simulink model "gm_parallel_8_prediction"  (R2022a)
settings: Solver=FixedStepDiscrete  StartTime=0.0  StopTime=10.0  RelTol=1e-3
undefined symbols (not defined in the file or in its folder): f_c, L_d, L_q, L_x, L_y, p, psi_pm, R_ph
libraries: hdlmdlgenlib x2
(part 1 of 4)
settings Model: Creator=Andre Merx  LastModifiedBy=Andre Merx
settings SolverCC: AlgebraicLoopSolver=TrustRegion
settings DataIOCC: LimitDataPoints=on  SaveOutput=off  SaveTime=off
settings OptimizationCC: BlockReduction=off  ConditionallyExecuteInputs=off  DefaultParameterBehavior=Inlined  LifeSpan=inf
settings DebuggingCC: AlgebraicLoopMsg=error  InheritedTsInSrcMsg=none  SingleTaskRateTransMsg=error  UnconnectedInputMsg=warning  UnconnectedOutputMsg=warning  UnconnectedLineMsg=warning  AllowSymbolicDim=off  StrictBusMsg=ErrorOnBusTreatedAsVector  SFUnexpectedBacktrackingDiag=warning  SFNoUnconditionalDefaultTransitionDiag=warning  SFExecutionAtInitializationDiag=none  SFMachineParentedDataDiag=warning  ArithmeticOperatorsInVariantConditions=warning
settings HardwareCC: ProdBitPerPointer=32  ProdBitPerSizeT=32  ProdBitPerPtrDiffT=32  ProdLargestAtomicFloat=None  ProdIntDivRoundTo=Undefined  ProdEndianess=Unspecified  ProdWordSize=32  ProdHWDeviceType=ASIC/FPGA->ASIC/FPGA  ProdEqTarget=off
settings SFSimCC: SimUseLocalCustomCode=off  CustomCodeUndefinedFunction=UseInterfaceOnly
settings RTWCC: RTWUseLocalCustomCode=off
settings CodeAppCC: StateflowObjectComments=on
settings GRTTargetCC: TargetLangStandard=C89/C90 (ANSI)
settings ConfigComp: CovScope=ReferencedModels  CovMetricSettings=dw  CovSaveCumulativeToWorkspaceVar=on  CovSaveSingleToWorkspaceVar=on  CovExternalEMLEnable=off  CovSFcnEnable=off

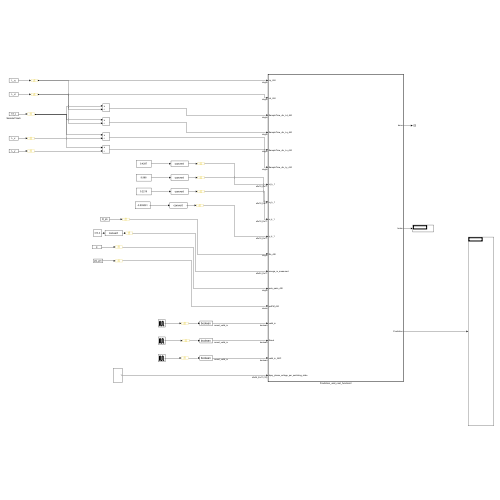
[thumbnail: Simulink's stored preview of the top-level diagram]
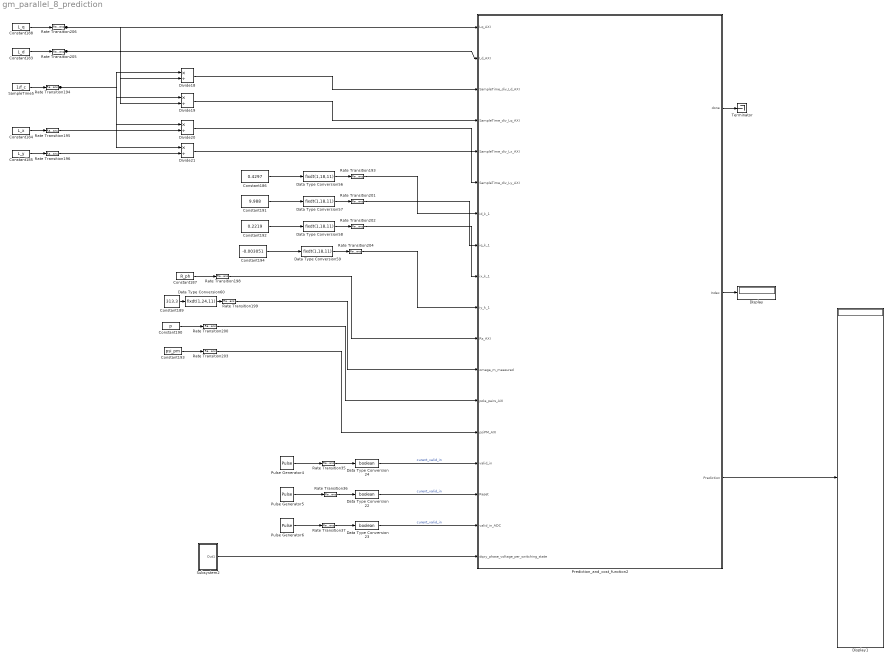
== system gm_parallel_8_prediction ==
  Constant183 : Constant  Value=L_d  OutDataTypeStr=single  SampleTime=-1
  Constant184 : Constant  Value=L_x  OutDataTypeStr=single  SampleTime=-1
  Constant185 : Constant  Value=L_y  OutDataTypeStr=single  SampleTime=-1
  Constant186 : Constant  Value=0.4297
  Constant187 : Constant  Value=R_ph  OutDataTypeStr=single  SampleTime=-1
  Constant188 : Constant  Value=L_q  OutDataTypeStr=single  SampleTime=-1
  Constant189 : Constant  Value=313.3
  Constant190 : Constant  Value=p  OutDataTypeStr=single  SampleTime=-1
  Constant191 : Constant  Value=9.988
  Constant192 : Constant  Value=0.2219
  Constant193 : Constant  Value=psi_pm  OutDataTypeStr=single  SampleTime=-1
  Constant194 : Constant  Value=-0.003051
  Data Type Conversion22 : DataTypeConversion  OutDataTypeStr=boolean  SaturateOnIntegerOverflow=off  RndMeth=Floor
  Data Type Conversion23 : DataTypeConversion  OutDataTypeStr=boolean  SaturateOnIntegerOverflow=off  RndMeth=Floor
  Data Type Conversion24 : DataTypeConversion  OutDataTypeStr=boolean  SaturateOnIntegerOverflow=off  RndMeth=Floor
  Data Type Conversion{56..59} (4 alike) : DataTypeConversion  OutDataTypeStr=fixdt(1,18,11)  SaturateOnIntegerOverflow=off  RndMeth=Floor
  Data Type Conversion60 : DataTypeConversion  OutDataTypeStr=fixdt(1,24,11)  SaturateOnIntegerOverflow=off  RndMeth=Floor
  Display : Display
  Display1 : Display
  Divide{18..21} (4 alike) : Product  Inputs=*/  RndMeth=Zero  SaturateOnIntegerOverflow=on
  Prediction_and_cost_function2 : Subsystem  TreatAsAtomicUnit=on
  Pulse Generator4 : DiscretePulseGenerator  PulseType=Time based  Period=1/f_c
  Pulse Generator5 : DiscretePulseGenerator  PulseType=Time based  Period=1/f_c
  Pulse Generator6 : DiscretePulseGenerator  PulseType=Time based  Period=1/f_c
  Rate Transition{35..37,193..196,198..206} (16 alike) : RateTransition  OutPortSampleTime=Rt
  SampleTime5 : Constant  Value=1/f_c  OutDataTypeStr=single  SampleTime=-1
  Subsystem2 : Subsystem
  Terminator : Terminator
  wires:
  Prediction_and_cost_function2/3(Prediction) -> Display1/1
  Prediction_and_cost_function2/2(Index) -> Display/1
  Prediction_and_cost_function2/1(done) -> Terminator/1
  Pulse Generator5/1 -> Rate Transition36/1
  Pulse Generator6/1 -> Rate Transition37/1
  Data Type Conversion22/1 -> Prediction_and_cost_function2/16(Reset)  "curent_valid_in"
  Data Type Conversion24/1 -> Prediction_and_cost_function2/15(valid_in)  "curent_valid_in"
  Rate Transition37/1 -> Data Type Conversion23/1
  Rate Transition35/1 -> Data Type Conversion24/1
  Data Type Conversion23/1 -> Prediction_and_cost_function2/17(valid_in_ADC)  "curent_valid_in"
  Rate Transition36/1 -> Data Type Conversion22/1
  Pulse Generator4/1 -> Rate Transition35/1
  Rate Transition204/1 -> Prediction_and_cost_function2/10(iy_k_1)
  Rate Transition193/1 -> Prediction_and_cost_function2/7(id_k_1)
  Rate Transition194/1 -> Divide18/1, Divide20/1, Divide21/1, Divide19/1
  Rate Transition198/1 -> Prediction_and_cost_function2/11(Rs_AXI)
  Divide18/1 -> Prediction_and_cost_function2/3(SampleTime_div_Ld_AXI)
  Constant191/1 -> Data Type Conversion57/1
  Constant185/1 -> Rate Transition196/1
  Rate Transition202/1 -> Prediction_and_cost_function2/9(ix_k_1)
  Divide21/1 -> Prediction_and_cost_function2/6(SampleTime_div_Ly_AXI)
  Constant189/1 -> Data Type Conversion60/1
  Constant183/1 -> Rate Transition205/1
  Constant184/1 -> Rate Transition195/1
  Constant193/1 -> Rate Transition203/1
  Rate Transition200/1 -> Prediction_and_cost_function2/13(pole_pairs_AXI)
  Rate Transition206/1 -> Prediction_and_cost_function2/1(Lq_AXI), Divide19/2
  Divide19/1 -> Prediction_and_cost_function2/4(SampleTime_div_Lq_AXI)
  Rate Transition196/1 -> Divide21/2
  Constant192/1 -> Data Type Conversion58/1
  Data Type Conversion56/1 -> Rate Transition193/1
  Rate Transition203/1 -> Prediction_and_cost_function2/14(psiPM_AXI)
  Constant187/1 -> Rate Transition198/1
  Divide20/1 -> Prediction_and_cost_function2/5(SampleTime_div_Lx_AXI)
  Data Type Conversion57/1 -> Rate Transition201/1
  Constant186/1 -> Data Type Conversion56/1
  SampleTime5/1 -> Rate Transition194/1
  Rate Transition195/1 -> Divide20/2
  Data Type Conversion58/1 -> Rate Transition202/1
  Rate Transition205/1 -> Prediction_and_cost_function2/2(Ld_AXI), Divide18/2
  Subsystem2/1(Out1) -> Prediction_and_cost_function2/18(dqxy_phase_voltage_per_switching_state)
  Constant190/1 -> Rate Transition200/1
  Data Type Conversion59/1 -> Rate Transition204/1
  Rate Transition201/1 -> Prediction_and_cost_function2/8(iq_k_1)
  Constant188/1 -> Rate Transition206/1
  Constant194/1 -> Data Type Conversion59/1
  Rate Transition199/1 -> Prediction_and_cost_function2/12(omega_m_measured)
  Data Type Conversion60/1 -> Rate Transition199/1

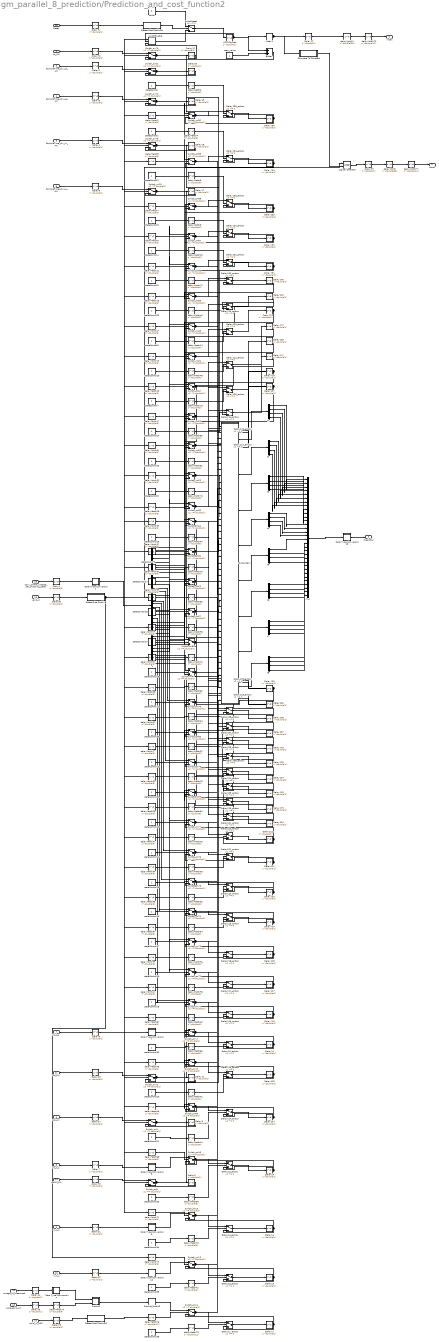
== system gm_parallel_8_prediction/Prediction_and_cost_function2 ==
  Lq_AXI : Inport  OutDataTypeStr=single  PortDimensions=1  SampleTime=1e-08
  Ld_AXI : Inport  Port=2  OutDataTypeStr=single  PortDimensions=1  SampleTime=1e-08
  SampleTime_div_Ld_AXI : Inport  Port=3  OutDataTypeStr=single  PortDimensions=1  SampleTime=1e-08
  SampleTime_div_Lq_AXI : Inport  Port=4  OutDataTypeStr=single  PortDimensions=1  SampleTime=1e-08
  SampleTime_div_Lx_AXI : Inport  Port=5  OutDataTypeStr=single  PortDimensions=1  SampleTime=1e-08
  SampleTime_div_Ly_AXI : Inport  Port=6  OutDataTypeStr=single  PortDimensions=1  SampleTime=1e-08
  id_k_1 : Inport  Port=7  OutDataTypeStr=fixdt(1, 18, 11)  PortDimensions=1  SampleTime=1e-08
  iq_k_1 : Inport  Port=8  OutDataTypeStr=fixdt(1, 18, 11)  PortDimensions=1  SampleTime=1e-08
  ix_k_1 : Inport  Port=9  OutDataTypeStr=fixdt(1, 18, 11)  PortDimensions=1  SampleTime=1e-08
  iy_k_1 : Inport  Port=10  OutDataTypeStr=fixdt(1, 18, 11)  PortDimensions=1  SampleTime=1e-08
  Rs_AXI : Inport  Port=11  OutDataTypeStr=single  PortDimensions=1  SampleTime=1e-08
  omega_m_measured : Inport  Port=12  OutDataTypeStr=fixdt(1, 24, 11)  PortDimensions=1  SampleTime=1e-08
  pole_pairs_AXI : Inport  Port=13  OutDataTypeStr=single  PortDimensions=1  SampleTime=1e-08
  psiPM_AXI : Inport  Port=14  OutDataTypeStr=single  PortDimensions=1  SampleTime=1e-08
  valid_in : Inport  Port=15  OutDataTypeStr=boolean  PortDimensions=1  SampleTime=1e-08
  Reset : Inport  Port=16  OutDataTypeStr=boolean  PortDimensions=1  SampleTime=1e-08
  valid_in_ADC : Inport  Port=17  OutDataTypeStr=boolean  PortDimensions=1  SampleTime=1e-08
  dqxy_phase_voltage_per_switching_state : Inport  Port=18  OutDataTypeStr=fixdt(1, 24, 11)  PortDimensions=[32]  SampleTime=1e-08
  Compare To Constant : Subsystem  mask(Compare To Constant){relop=<=, const=double(8), OutDataTypeStr=boolean, ZeroCross=on}
      mask prompts: relop "Simulink:masks:Operator_MP"; const "Simulink:masks:ConstantValue_MP"; OutDataTypeStr "Simulink:masks:OutputDataType_MP"; ZeroCross "Simulink:masks:EnableZerocrossingDetection_MP"
      mask help: Simulink:masks:CompareToConstant_MD
      mask init:
      | OutDataTypeStr = 'boolean';
      | ZeroCross = 'on';
      | blkName = 'parallel_8_prediction/Prediction_and_cost_function2/Compare\nTo Constant';
      | const = double(8);
      | const_str = '8';
      | const_val = double(8);
      | relop = '<=';
      | setValue = 'boolean';
      | str = '<= 8';
      mask TypeOptions relop: == | ~= | < | <= | >= | >
      mask TypeOptions OutDataTypeStr: Simulink:masks:uint8 | Simulink:masks:boolean
      mask Callback ZeroCross: sl('zeroCrossEnable', gcbh);
      mask Display: disp(str)
  Data Type Conversion1 : Subsystem
      mask Display: disp('NFP\nconv');
  Data Type Conversion10 : Subsystem
      mask Display: disp('NFP\nconv');
  Data Type Conversion18 : Subsystem
      mask Display: disp('NFP\nconv');
  Data Type Conversion4 : Subsystem
      mask Display: disp('NFP\nconv');
  Data Type Conversion7 : Subsystem
      mask Display: disp('NFP\nconv');
  Data Type Conversion8 : Subsystem
      mask Display: disp('NFP\nconv');
  Data Type Conversion9 : Subsystem
      mask Display: disp('NFP\nconv');
  Delay{1..33,104..135} (65 alike) : Delay  DelayLength=double(1)  InitialCondition=0  SampleTime=1e-08
  Delay104_enbsw : Switch  Criteria=u2 ~= 0  Threshold=double(0)  OutDataTypeStr=single  SampleTime=1e-08  SaturateOnIntegerOverflow=off  InputSameDT=off
  Delay105_enbsw : Switch  Criteria=u2 ~= 0  Threshold=double(0)  OutDataTypeStr=single  SampleTime=1e-08  SaturateOnIntegerOverflow=off  InputSameDT=off
  Delay106_enbsw : Switch  Criteria=u2 ~= 0  Threshold=double(0)  OutDataTypeStr=single  SampleTime=1e-08  SaturateOnIntegerOverflow=off  InputSameDT=off
  Delay107_enbsw : Switch  Criteria=u2 ~= 0  Threshold=double(0)  OutDataTypeStr=single  SampleTime=1e-08  SaturateOnIntegerOverflow=off  InputSameDT=off
  Delay108_enbsw : Switch  Criteria=u2 ~= 0  Threshold=double(0)  OutDataTypeStr=single  SampleTime=1e-08  SaturateOnIntegerOverflow=off  InputSameDT=off
  Delay109_enbsw : Switch  Criteria=u2 ~= 0  Threshold=double(0)  OutDataTypeStr=single  SampleTime=1e-08  SaturateOnIntegerOverflow=off  InputSameDT=off
  Delay110_enbsw : Switch  Criteria=u2 ~= 0  Threshold=double(0)  OutDataTypeStr=single  SampleTime=1e-08  SaturateOnIntegerOverflow=off  InputSameDT=off
  Delay111_enbsw : Switch  Criteria=u2 ~= 0  Threshold=double(0)  OutDataTypeStr=single  SampleTime=1e-08  SaturateOnIntegerOverflow=off  InputSameDT=off
  Delay112_enbsw : Switch  Criteria=u2 ~= 0  Threshold=double(0)  OutDataTypeStr=single  SampleTime=1e-08  SaturateOnIntegerOverflow=off  InputSameDT=off
  Delay113_enbsw : Switch  Criteria=u2 ~= 0  Threshold=double(0)  OutDataTypeStr=single  SampleTime=1e-08  SaturateOnIntegerOverflow=off  InputSameDT=off
  Delay114_enbsw : Switch  Criteria=u2 ~= 0  Threshold=double(0)  OutDataTypeStr=single  SampleTime=1e-08  SaturateOnIntegerOverflow=off  InputSameDT=off
  Delay115_enbsw : Switch  Criteria=u2 ~= 0  Threshold=double(0)  OutDataTypeStr=single  SampleTime=1e-08  SaturateOnIntegerOverflow=off  InputSameDT=off
  Delay116_enbsw : Switch  Criteria=u2 ~= 0  Threshold=double(0)  OutDataTypeStr=single  SampleTime=1e-08  SaturateOnIntegerOverflow=off  InputSameDT=off
  Delay117_enbsw : Switch  Criteria=u2 ~= 0  Threshold=double(0)  OutDataTypeStr=single  SampleTime=1e-08  SaturateOnIntegerOverflow=off  InputSameDT=off
  Delay118_enbsw : Switch  Criteria=u2 ~= 0  Threshold=double(0)  OutDataTypeStr=single  SampleTime=1e-08  SaturateOnIntegerOverflow=off  InputSameDT=off
  Delay119_enbsw : Switch  Criteria=u2 ~= 0  Threshold=double(0)  OutDataTypeStr=single  SampleTime=1e-08  SaturateOnIntegerOverflow=off  InputSameDT=off
  Delay11_enbsw : Switch  Criteria=u2 ~= 0  Threshold=double(0)  OutDataTypeStr=single  SampleTime=1e-08  SaturateOnIntegerOverflow=off  InputSameDT=off
  Delay120_enbsw : Switch  Criteria=u2 ~= 0  Threshold=double(0)  OutDataTypeStr=single  SampleTime=1e-08  SaturateOnIntegerOverflow=off  InputSameDT=off
  Delay121_enbsw : Switch  Criteria=u2 ~= 0  Threshold=double(0)  OutDataTypeStr=single  SampleTime=1e-08  SaturateOnIntegerOverflow=off  InputSameDT=off
  Delay122_enbsw : Switch  Criteria=u2 ~= 0  Threshold=double(0)  OutDataTypeStr=single  SampleTime=1e-08  SaturateOnIntegerOverflow=off  InputSameDT=off
  Delay123_enbsw : Switch  Criteria=u2 ~= 0  Threshold=double(0)  OutDataTypeStr=single  SampleTime=1e-08  SaturateOnIntegerOverflow=off  InputSameDT=off
  Delay124_enbsw : Switch  Criteria=u2 ~= 0  Threshold=double(0)  OutDataTypeStr=single  SampleTime=1e-08  SaturateOnIntegerOverflow=off  InputSameDT=off
  Delay125_enbsw : Switch  Criteria=u2 ~= 0  Threshold=double(0)  OutDataTypeStr=single  SampleTime=1e-08  SaturateOnIntegerOverflow=off  InputSameDT=off
  Delay126_enbsw : Switch  Criteria=u2 ~= 0  Threshold=double(0)  OutDataTypeStr=single  SampleTime=1e-08  SaturateOnIntegerOverflow=off  InputSameDT=off
  Delay127_enbsw : Switch  Criteria=u2 ~= 0  Threshold=double(0)  OutDataTypeStr=single  SampleTime=1e-08  SaturateOnIntegerOverflow=off  InputSameDT=off
  Delay128_enbsw : Switch  Criteria=u2 ~= 0  Threshold=double(0)  OutDataTypeStr=single  SampleTime=1e-08  SaturateOnIntegerOverflow=off  InputSameDT=off
  Delay129_enbsw : Switch  Criteria=u2 ~= 0  Threshold=double(0)  OutDataTypeStr=single  SampleTime=1e-08  SaturateOnIntegerOverflow=off  InputSameDT=off
  Delay130_enbsw : Switch  Criteria=u2 ~= 0  Threshold=double(0)  OutDataTypeStr=single  SampleTime=1e-08  SaturateOnIntegerOverflow=off  InputSameDT=off
  Delay131_enbsw : Switch  Criteria=u2 ~= 0  Threshold=double(0)  OutDataTypeStr=single  SampleTime=1e-08  SaturateOnIntegerOverflow=off  InputSameDT=off
  Delay132_enbsw : Switch  Criteria=u2 ~= 0  Threshold=double(0)  OutDataTypeStr=single  SampleTime=1e-08  SaturateOnIntegerOverflow=off  InputSameDT=off
  Delay133_enbsw : Switch  Criteria=u2 ~= 0  Threshold=double(0)  OutDataTypeStr=single  SampleTime=1e-08  SaturateOnIntegerOverflow=off  InputSameDT=off
  Delay134_enbsw : Switch  Criteria=u2 ~= 0  Threshold=double(0)  OutDataTypeStr=single  SampleTime=1e-08  SaturateOnIntegerOverflow=off  InputSameDT=off
  Delay135_enbsw : Switch  Criteria=u2 ~= 0  Threshold=double(0)  OutDataTypeStr=single  SampleTime=1e-08  SaturateOnIntegerOverflow=off  InputSameDT=off
  Delay13_enbsw : Switch  Criteria=u2 ~= 0  Threshold=double(0)  OutDataTypeStr=single  SampleTime=1e-08  SaturateOnIntegerOverflow=off  InputSameDT=off
  Delay14_enbsw : Switch  Criteria=u2 ~= 0  Threshold=double(0)  OutDataTypeStr=single  SampleTime=1e-08  SaturateOnIntegerOverflow=off  InputSameDT=off
  Delay15_enbsw : Switch  Criteria=u2 ~= 0  Threshold=double(0)  OutDataTypeStr=single  SampleTime=1e-08  SaturateOnIntegerOverflow=off  InputSameDT=off
  Delay16_enbsw : Switch  Criteria=u2 ~= 0  Threshold=double(0)  OutDataTypeStr=single  SampleTime=1e-08  SaturateOnIntegerOverflow=off  InputSameDT=off
  Detect Rise Positive : Subsystem  mask(Detect Rise Positive){vinit=double(0), InputProcessing=Elements as channels (sample based), OutDataTypeStr=boolean}
      mask prompts: vinit "Simulink:masks:InitialCondition_MP"; InputProcessing "Simulink:masks:InputProcessing_MP"; OutDataTypeStr "Simulink:masks:OutputDataType_MP"
      mask help: Simulink:masks:DetectRisePositive_MD
      mask init:
      | InputProcessing = 'Elements as channels (sample based)';
      | OutDataTypeStr = 'boolean';
      | vinit = double(0);
      mask TypeOptions InputProcessing: Simulink:masks:ColumnsAsChannelsFrameBased | Simulink:masks:ElementsAsChannelsSampleBased
      mask TypeOptions OutDataTypeStr: Simulink:masks:uint8 | Simulink:masks:boolean
      mask Display: fprintf('U > 0\n&  NOT\nU/z > 0')
  Detect Rise Positive1 : Subsystem  mask(Detect Rise Positive){vinit=double(0), InputProcessing=Elements as channels (sample based), OutDataTypeStr=boolean}
      mask prompts: vinit "Simulink:masks:InitialCondition_MP"; InputProcessing "Simulink:masks:InputProcessing_MP"; OutDataTypeStr "Simulink:masks:OutputDataType_MP"
      mask help: Simulink:masks:DetectRisePositive_MD
      mask init:
      | InputProcessing = 'Elements as channels (sample based)';
      | OutDataTypeStr = 'boolean';
      | vinit = double(0);
      mask TypeOptions InputProcessing: Simulink:masks:ColumnsAsChannelsFrameBased | Simulink:masks:ElementsAsChannelsSampleBased
      mask TypeOptions OutDataTypeStr: Simulink:masks:uint8 | Simulink:masks:boolean
      mask Display: fprintf('U > 0\n&  NOT\nU/z > 0')
  Detect Rise Positive2 : Subsystem  mask(Detect Rise Positive){vinit=double(0), InputProcessing=Elements as channels (sample based), OutDataTypeStr=boolean}
      mask prompts: vinit "Simulink:masks:InitialCondition_MP"; InputProcessing "Simulink:masks:InputProcessing_MP"; OutDataTypeStr "Simulink:masks:OutputDataType_MP"
      mask help: Simulink:masks:DetectRisePositive_MD
      mask init:
      | InputProcessing = 'Elements as channels (sample based)';
      | OutDataTypeStr = 'boolean';
      | vinit = double(0);
      mask TypeOptions InputProcessing: Simulink:masks:ColumnsAsChannelsFrameBased | Simulink:masks:ElementsAsChannelsSampleBased
      mask TypeOptions OutDataTypeStr: Simulink:masks:uint8 | Simulink:masks:boolean
      mask Display: fprintf('U > 0\n&  NOT\nU/z > 0')
  HDL Counter : Delay  DelayLength=double(1)  InitialCondition=0  SampleTime=1e-08
  Index1 : hdlmdlgenlib/Buffer
      settings: SourceProductBaseCode=SL
  Logical Operator : Logic  AllPortsSameDT=off  OutDataTypeStr=boolean  SampleTime=1e-08
  Product : Subsystem
      mask Display: disp('NFP\nmul');
  Product_outbuff : hdlmdlgenlib/Buffer
      settings: SourceProductBaseCode=SL
  Subsystem : Subsystem
  Switch_on{8..13,15..21,59..90} (45 alike) : Switch  Threshold=double(1)  OutDataTypeStr=single  RndMeth=Simplest  SampleTime=1e-08  SaturateOnIntegerOverflow=off  InputSameDT=off
  adder : Sum  AccumDataTypeStr=int32  OutDataTypeStr=int32  SampleTime=1e-08
  const : Constant  Value=0  VectorParams1D=off  OutDataTypeStr=int32  SampleTime=1e-08
  delayMatch : Delay  DelayLength=double(36)  InitialCondition=0  SampleTime=1e-08
  delayMatch1 : Delay  DelayLength=double(36)  InitialCondition=0  SampleTime=1e-08
  delayMatch{2..74} (73 alike) : Delay  DelayLength=double(6)  InitialCondition=0  SampleTime=1e-08
  delayMatch75 : Delay  DelayLength=double(12)  InitialCondition=0  SampleTime=1e-08
  delayMatch76 : Delay  DelayLength=double(12)  InitialCondition=0  SampleTime=1e-08
  delayMatch77 : Delay  DelayLength=double(11)  InitialCondition=0  SampleTime=1e-08
  delayMatch78 : Delay  DelayLength=double(11)  InitialCondition=0  SampleTime=1e-08
  mux : Mux  Inputs=32
  stateControl{,1..36} (37 alike) : Constant  OutDataTypeStr=boolean  SampleTime=1e-08
  step_value : Constant  VectorParams1D=off  OutDataTypeStr=int32  SampleTime=1e-08
  switchEnable : MultiPortSwitch  DataPortOrder=Zero-based contiguous  Inputs=2  DiagnosticForDefault=None  zeroidx=on  OutDataTypeStr=int32  SampleTime=1e-08  SaturateOnIntegerOverflow=off  InputSameDT=off
  switchReset : Switch  Criteria=u2 ~= 0  Threshold=double(0)  OutDataTypeStr=int32  SampleTime=1e-08  SaturateOnIntegerOverflow=off  InputSameDT=off
  t : Demux  Outputs=32
  t{1..8} (8 alike) : Demux
  done : Outport  SampleTime=1e-08
  Index : Outport  Port=2  SampleTime=1e-08
  Prediction : Outport  Port=3  SampleTime=1e-08
  wires:
  Lq_AXI/1 -> Delay26/1
  Ld_AXI/1 -> Delay27/1
  SampleTime_div_Ld_AXI/1 -> Delay2/1
  SampleTime_div_Lq_AXI/1 -> Delay3/1
  SampleTime_div_Lx_AXI/1 -> Delay4/1
  SampleTime_div_Ly_AXI/1 -> Delay5/1
  id_k_1/1 -> Delay6/1
  iq_k_1/1 -> Delay7/1
  ix_k_1/1 -> Delay21/1
  iy_k_1/1 -> Delay22/1
  Rs_AXI/1 -> Delay23/1
  omega_m_measured/1 -> Delay24/1
  pole_pairs_AXI/1 -> Delay25/1
  psiPM_AXI/1 -> Delay28/1
  valid_in/1 -> Delay30/1
  Reset/1 -> Delay31/1
  valid_in_ADC/1 -> Delay29/1
  dqxy_phase_voltage_per_switching_state/1 -> Delay1/1
  Compare To Constant/1(y) -> Logical Operator/2
  Delay1/1 -> Data Type Conversion1/1(In1)
  Delay2/1 -> Switch_on21/1
  Delay21/1 -> Data Type Conversion9/1(In1)
  Delay22/1 -> Data Type Conversion10/1(In1)
  Delay23/1 -> Switch_on12/1
  Delay24/1 -> Data Type Conversion4/1(In1)
  delayMatch74/1 -> Product/2(In2)
  Delay26/1 -> Switch_on10/1
  Delay27/1 -> Switch_on9/1
  Delay28/1 -> Switch_on8/1
  Delay29/1 -> Detect Rise Positive2/1(U)
  Delay3/1 -> Switch_on20/1
  Delay30/1 -> Detect Rise Positive/1(U)
  Delay31/1 -> Detect Rise Positive1/1(U)
  delayMatch78/1 -> Index/1
  delayMatch77/1 -> done/1
  Delay4/1 -> Switch_on19/1
  Delay5/1 -> Switch_on18/1
  Delay6/1 -> Data Type Conversion7/1(In1)
  Delay7/1 -> Data Type Conversion8/1(In1)
  delayMatch3/1 -> Switch_on90/2
  Detect Rise Positive1/1(Y) -> switchReset/2
  delayMatch76/1 -> Switch_on11/2
  Index1/1 -> Delay32/1, Compare To Constant/1(u)
  Logical Operator/1 -> Delay33/1
  mux/1 -> Data Type Conversion18/1(In1)
  Product_outbuff/1 -> Switch_on11/1
  Subsystem/1(Prediction_1) -> t1/1
  Subsystem/2(Prediction_2) -> t2/1
  Subsystem/3(Prediction_3) -> t3/1
  Subsystem/4(Prediction_4) -> t4/1
  Subsystem/5(Prediction_5) -> t5/1
  Subsystem/6(Prediction_6) -> t6/1
  Subsystem/7(Prediction_7) -> t7/1
  Subsystem/8(Prediction_8) -> t8/1
  Switch_on10/1 -> Subsystem/43(Lq15), Delay10/1
  Switch_on12/1 -> Subsystem/41(Rs15), Delay12/1
  Switch_on18/1 -> Subsystem/36(SampleTime_div_Ly15), Delay17/1
  Switch_on19/1 -> Subsystem/35(SampleTime_div_Lx15), Delay18/1
  Switch_on20/1 -> Subsystem/34(SampleTime_div_Lq15), Delay19/1
  Switch_on21/1 -> Subsystem/33(SampleTime_div_Ld15), Delay20/1
  Switch_on8/1 -> Subsystem/45(psiPM15), Delay8/1
  Switch_on9/1 -> Subsystem/44(Ld15), Delay9/1
  HDL Counter/1 -> Index1/1, switchEnable/2, adder/1
  const/1 -> switchReset/1
  step_value/1 -> adder/2
  t/1 -> Switch_on90/1
  t/2 -> Switch_on89/1
  t/3 -> Switch_on88/1
  t/4 -> Switch_on87/1
  t/5 -> Switch_on86/1
  t/6 -> Switch_on85/1
  t/7 -> Switch_on84/1
  t/8 -> Switch_on83/1
  t/9 -> Switch_on82/1
  t/10 -> Switch_on81/1
  t/11 -> Switch_on80/1
  t/12 -> Switch_on79/1
  t/13 -> Switch_on78/1
  t/14 -> Switch_on77/1
  t/15 -> Switch_on76/1
  t/16 -> Switch_on75/1
  t/17 -> Switch_on74/1
  t/18 -> Switch_on73/1
  t/19 -> Switch_on72/1
  t/20 -> Switch_on71/1
  t/21 -> Switch_on70/1
  t/22 -> Switch_on69/1
  t/23 -> Switch_on68/1
  t/24 -> Switch_on67/1
  t/25 -> Switch_on66/1
  t/26 -> Switch_on65/1
  t/27 -> Switch_on64/1
  t/28 -> Switch_on63/1
  t/29 -> Switch_on62/1
  t/30 -> Switch_on61/1
  t/31 -> Switch_on60/1
  t/32 -> Switch_on59/1
  t1/1 -> mux/1
  t1/2 -> mux/2
  t1/3 -> mux/3
  t1/4 -> mux/4
  t2/1 -> mux/5
  t2/2 -> mux/6
  t2/3 -> mux/7
  t2/4 -> mux/8
  t3/1 -> mux/9
  t3/2 -> mux/10
  t3/3 -> mux/11
  t3/4 -> mux/12
  t4/1 -> mux/13
  t4/2 -> mux/14
  t4/3 -> mux/15
  t4/4 -> mux/16
  t5/1 -> mux/17
  t5/2 -> mux/18
  t5/3 -> mux/19
  t5/4 -> mux/20
  t6/1 -> mux/21
  t6/2 -> mux/22
  t6/3 -> mux/23
  t6/4 -> mux/24
  t7/1 -> mux/25
  t7/2 -> mux/26
  t7/3 -> mux/27
  t7/4 -> mux/28
  t8/1 -> mux/29
  t8/2 -> mux/30
  t8/3 -> mux/31
  t8/4 -> mux/32
  Delay33/1 -> delayMatch/1
  Delay32/1 -> delayMatch1/1
  Data Type Conversion1/1(Out1) -> t/1
  Data Type Conversion10/1(Out1) -> Switch_on13/1
  Data Type Conversion18/1(Out1) -> Prediction/1
  Data Type Conversion4/1(Out1) -> Product/1(In1)
  Data Type Conversion7/1(Out1) -> Switch_on17/1
  Data Type Conversion8/1(Out1) -> Switch_on16/1
  Data Type Conversion9/1(Out1) -> Switch_on15/1
  Product/1(Out1) -> Product_outbuff/1
  delayMatch2/1 -> Delay135_enbsw/2
  delayMatch4/1 -> Delay134_enbsw/2
  delayMatch6/1 -> Delay133_enbsw/2
  delayMatch8/1 -> Delay132_enbsw/2
  delayMatch10/1 -> Delay131_enbsw/2
  delayMatch12/1 -> Delay130_enbsw/2
  delayMatch14/1 -> Delay129_enbsw/2
  delayMatch16/1 -> Delay128_enbsw/2
  delayMatch18/1 -> Delay127_enbsw/2
  delayMatch20/1 -> Delay126_enbsw/2
  delayMatch22/1 -> Delay125_enbsw/2
  delayMatch24/1 -> Delay124_enbsw/2
  delayMatch26/1 -> Delay123_enbsw/2
  delayMatch28/1 -> Delay122_enbsw/2
  delayMatch30/1 -> Delay121_enbsw/2
  delayMatch32/1 -> Delay120_enbsw/2
  delayMatch34/1 -> Delay119_enbsw/2
  delayMatch36/1 -> Delay118_enbsw/2
  delayMatch38/1 -> Delay117_enbsw/2
  delayMatch40/1 -> Delay116_enbsw/2
  delayMatch42/1 -> Delay115_enbsw/2
  delayMatch44/1 -> Delay114_enbsw/2
  delayMatch46/1 -> Delay113_enbsw/2
  delayMatch48/1 -> Delay112_enbsw/2
  delayMatch50/1 -> Delay111_enbsw/2
  delayMatch52/1 -> Delay110_enbsw/2
  delayMatch54/1 -> Delay109_enbsw/2
  delayMatch56/1 -> Delay108_enbsw/2
  delayMatch58/1 -> Delay107_enbsw/2
  delayMatch60/1 -> Delay106_enbsw/2
  delayMatch62/1 -> Delay105_enbsw/2
  delayMatch64/1 -> Delay104_enbsw/2
  delayMatch66/1 -> Delay16_enbsw/2
  delayMatch68/1 -> Delay15_enbsw/2
  delayMatch70/1 -> Delay14_enbsw/2
  delayMatch72/1 -> Delay13_enbsw/2
  delayMatch75/1 -> Delay11_enbsw/2
  stateControl/1 -> delayMatch2/1
  delayMatch5/1 -> Switch_on89/2
  stateControl1/1 -> delayMatch4/1
  delayMatch7/1 -> Switch_on88/2
  stateControl2/1 -> delayMatch6/1
  delayMatch9/1 -> Switch_on87/2
  stateControl3/1 -> delayMatch8/1
  delayMatch11/1 -> Switch_on86/2
  stateControl4/1 -> delayMatch10/1
  delayMatch13/1 -> Switch_on85/2
  stateControl5/1 -> delayMatch12/1
  delayMatch15/1 -> Switch_on84/2
  stateControl6/1 -> delayMatch14/1
  delayMatch17/1 -> Switch_on83/2
  stateControl7/1 -> delayMatch16/1
  delayMatch19/1 -> Switch_on82/2
  stateControl8/1 -> delayMatch18/1
  delayMatch21/1 -> Switch_on81/2
  stateControl9/1 -> delayMatch20/1
  delayMatch23/1 -> Switch_on80/2
  stateControl10/1 -> delayMatch22/1
  delayMatch25/1 -> Switch_on79/2
  stateControl11/1 -> delayMatch24/1
  delayMatch27/1 -> Switch_on78/2
  stateControl12/1 -> delayMatch26/1
  delayMatch29/1 -> Switch_on77/2
  stateControl13/1 -> delayMatch28/1
  delayMatch31/1 -> Switch_on76/2
  stateControl14/1 -> delayMatch30/1
  delayMatch33/1 -> Switch_on75/2
  stateControl15/1 -> delayMatch32/1
  delayMatch35/1 -> Switch_on74/2
  stateControl16/1 -> delayMatch34/1
  delayMatch37/1 -> Switch_on73/2
  stateControl17/1 -> delayMatch36/1
  delayMatch39/1 -> Switch_on72/2
  stateControl18/1 -> delayMatch38/1
  delayMatch41/1 -> Switch_on71/2
  stateControl19/1 -> delayMatch40/1
  delayMatch43/1 -> Switch_on70/2
  stateControl20/1 -> delayMatch42/1
  delayMatch45/1 -> Switch_on69/2
  stateControl21/1 -> delayMatch44/1
  delayMatch47/1 -> Switch_on68/2
  stateControl22/1 -> delayMatch46/1
  delayMatch49/1 -> Switch_on67/2
  stateControl23/1 -> delayMatch48/1
  delayMatch51/1 -> Switch_on66/2
  stateControl24/1 -> delayMatch50/1
  delayMatch53/1 -> Switch_on65/2
  stateControl25/1 -> delayMatch52/1
  delayMatch55/1 -> Switch_on64/2
  stateControl26/1 -> delayMatch54/1
  delayMatch57/1 -> Switch_on63/2
  stateControl27/1 -> delayMatch56/1
  delayMatch59/1 -> Switch_on62/2
  stateControl28/1 -> delayMatch58/1
  delayMatch61/1 -> Switch_on61/2
  stateControl29/1 -> delayMatch60/1
  delayMatch63/1 -> Switch_on60/2
  stateControl30/1 -> delayMatch62/1
  delayMatch65/1 -> Switch_on59/2
  stateControl31/1 -> delayMatch64/1
  delayMatch67/1 -> Switch_on17/2
  stateControl32/1 -> delayMatch66/1
  delayMatch69/1 -> Switch_on16/2
  stateControl33/1 -> delayMatch68/1
  delayMatch71/1 -> Switch_on15/2
  stateControl34/1 -> delayMatch70/1
  delayMatch73/1 -> Switch_on13/2
  stateControl35/1 -> delayMatch72/1
  Detect Rise Positive/1(Y) -> delayMatch73/1, delayMatch71/1, delayMatch69/1, delayMatch67/1, delayMatch65/1, delayMatch63/1, delayMatch61/1, delayMatch59/1, delayMatch57/1, delayMatch55/1, delayMatch53/1, delayMatch51/1, delayMatch49/1, delayMatch47/1, delayMatch45/1, delayMatch43/1, delayMatch41/1, delayMatch39/1, delayMatch37/1, delayMatch35/1, delayMatch33/1, delayMatch31/1, delayMatch29/1, delayMatch27/1, delayMatch25/1, delayMatch23/1, delayMatch21/1, delayMatch19/1, delayMatch17/1, delayMatch15/1, delayMatch13/1, delayMatch11/1, delayMatch9/1, delayMatch7/1, delayMatch5/1, delayMatch3/1, Logical Operator/1, switchEnable/1, Switch_on21/2, Switch_on20/2, Switch_on19/2, Switch_on18/2, Switch_on12/2, Switch_on10/2, Switch_on9/2, Switch_on8/2
  Delay25/1 -> delayMatch74/1
  stateControl36/1 -> delayMatch75/1
  Detect Rise Positive2/1(Y) -> delayMatch76/1
  delayMatch/1 -> delayMatch77/1
  delayMatch1/1 -> delayMatch78/1
  Switch_on90/1 -> Subsystem/1(d_phase_voltage_per_switching_state), Delay135_enbsw/1
  Switch_on89/1 -> Subsystem/2(q_phase_voltage_per_switching_state), Delay134_enbsw/1
  Switch_on88/1 -> Subsystem/3(x_phase_voltage_per_switching_state), Delay133_enbsw/1
  Switch_on87/1 -> Subsystem/4(y_phase_voltage_per_switching_state), Delay132_enbsw/1
  Switch_on86/1 -> Subsystem/5(d_phase_voltage_per_switching_state1), Delay131_enbsw/1
  Switch_on85/1 -> Subsystem/6(q_phase_voltage_per_switching_state1), Delay130_enbsw/1
  Switch_on84/1 -> Subsystem/7(x_phase_voltage_per_switching_state1), Delay129_enbsw/1
  Switch_on83/1 -> Subsystem/8(y_phase_voltage_per_switching_state1), Delay128_enbsw/1
  Switch_on82/1 -> Subsystem/9(d_phase_voltage_per_switching_state2), Delay127_enbsw/1
  Switch_on81/1 -> Subsystem/10(q_phase_voltage_per_switching_state2), Delay126_enbsw/1
  Switch_on80/1 -> Subsystem/11(x_phase_voltage_per_switching_state2), Delay125_enbsw/1
  Switch_on79/1 -> Subsystem/12(y_phase_voltage_per_switching_state2), Delay124_enbsw/1
  Switch_on78/1 -> Subsystem/13(d_phase_voltage_per_switching_state3), Delay123_enbsw/1
  Switch_on77/1 -> Subsystem/14(q_phase_voltage_per_switching_state3), Delay122_enbsw/1
  Switch_on76/1 -> Subsystem/15(x_phase_voltage_per_switching_state3), Delay121_enbsw/1
  Switch_on75/1 -> Subsystem/16(y_phase_voltage_per_switching_state3), Delay120_enbsw/1
  Switch_on74/1 -> Subsystem/17(d_phase_voltage_per_switching_state4), Delay119_enbsw/1
  Switch_on73/1 -> Subsystem/18(q_phase_voltage_per_switching_state4), Delay118_enbsw/1
  Switch_on72/1 -> Subsystem/19(x_phase_voltage_per_switching_state4), Delay117_enbsw/1
  Switch_on71/1 -> Subsystem/20(y_phase_voltage_per_switching_state4), Delay116_enbsw/1
  Switch_on70/1 -> Subsystem/21(d_phase_voltage_per_switching_state5), Delay115_enbsw/1
  Switch_on69/1 -> Subsystem/22(q_phase_voltage_per_switching_state5), Delay114_enbsw/1
  Switch_on68/1 -> Subsystem/23(x_phase_voltage_per_switching_state5), Delay113_enbsw/1
  Switch_on67/1 -> Subsystem/24(y_phase_voltage_per_switching_state5), Delay112_enbsw/1
  Switch_on66/1 -> Subsystem/25(d_phase_voltage_per_switching_state6), Delay111_enbsw/1
  Switch_on65/1 -> Subsystem/26(q_phase_voltage_per_switching_state6), Delay110_enbsw/1
  Switch_on64/1 -> Subsystem/27(x_phase_voltage_per_switching_state6), Delay109_enbsw/1
  Switch_on63/1 -> Subsystem/28(y_phase_voltage_per_switching_state6), Delay108_enbsw/1
  Switch_on62/1 -> Subsystem/29(d_phase_voltage_per_switching_state7), Delay107_enbsw/1
  Switch_on61/1 -> Subsystem/30(q_phase_voltage_per_switching_state7), Delay106_enbsw/1
  Switch_on60/1 -> Subsystem/31(x_phase_voltage_per_switching_state7), Delay105_enbsw/1
  Switch_on59/1 -> Subsystem/32(y_phase_voltage_per_switching_state7), Delay104_enbsw/1
  Switch_on17/1 -> Subsystem/37(id_k_16), Delay16_enbsw/1
  Switch_on16/1 -> Subsystem/38(iq_k_16), Delay15_enbsw/1
  Switch_on15/1 -> Subsystem/39(ix_k_16), Delay14_enbsw/1
  Switch_on13/1 -> Subsystem/40(iy_k_16), Delay13_enbsw/1
  Switch_on11/1 -> Subsystem/42(omega_el15), Delay11_enbsw/1
  adder/1 -> switchEnable/3
  switchEnable/1 -> switchReset/3
  switchReset/1 -> HDL Counter/1
  Delay135_enbsw/1 -> Delay135/1
  Delay135/1 -> Switch_on90/3, Delay135_enbsw/3
  Delay134_enbsw/1 -> Delay134/1
  Delay134/1 -> Switch_on89/3, Delay134_enbsw/3
  Delay133_enbsw/1 -> Delay133/1
  Delay133/1 -> Switch_on88/3, Delay133_enbsw/3
  Delay132_enbsw/1 -> Delay132/1
  Delay132/1 -> Switch_on87/3, Delay132_enbsw/3
  Delay131_enbsw/1 -> Delay131/1
  Delay131/1 -> Switch_on86/3, Delay131_enbsw/3
  Delay130_enbsw/1 -> Delay130/1
  Delay130/1 -> Switch_on85/3, Delay130_enbsw/3
  Delay129_enbsw/1 -> Delay129/1
  Delay129/1 -> Switch_on84/3, Delay129_enbsw/3
  Delay128_enbsw/1 -> Delay128/1
  Delay128/1 -> Switch_on83/3, Delay128_enbsw/3
  Delay127_enbsw/1 -> Delay127/1
  Delay127/1 -> Switch_on82/3, Delay127_enbsw/3
  Delay126_enbsw/1 -> Delay126/1
  Delay126/1 -> Switch_on81/3, Delay126_enbsw/3
  Delay125_enbsw/1 -> Delay125/1
  Delay125/1 -> Switch_on80/3, Delay125_enbsw/3
  Delay124_enbsw/1 -> Delay124/1
  Delay124/1 -> Switch_on79/3, Delay124_enbsw/3
  Delay123_enbsw/1 -> Delay123/1
  Delay123/1 -> Switch_on78/3, Delay123_enbsw/3
  Delay122_enbsw/1 -> Delay122/1
  Delay122/1 -> Switch_on77/3, Delay122_enbsw/3
  Delay121_enbsw/1 -> Delay121/1
  Delay121/1 -> Switch_on76/3, Delay121_enbsw/3
  Delay120_enbsw/1 -> Delay120/1
  Delay120/1 -> Switch_on75/3, Delay120_enbsw/3
  Delay119_enbsw/1 -> Delay119/1
  Delay119/1 -> Switch_on74/3, Delay119_enbsw/3
  Delay118_enbsw/1 -> Delay118/1
  Delay118/1 -> Switch_on73/3, Delay118_enbsw/3
  Delay117_enbsw/1 -> Delay117/1
  Delay117/1 -> Switch_on72/3, Delay117_enbsw/3
  Delay116_enbsw/1 -> Delay116/1
  Delay116/1 -> Switch_on71/3, Delay116_enbsw/3
  Delay115_enbsw/1 -> Delay115/1
  Delay115/1 -> Switch_on70/3, Delay115_enbsw/3
  Delay114_enbsw/1 -> Delay114/1
  Delay114/1 -> Switch_on69/3, Delay114_enbsw/3
  Delay113_enbsw/1 -> Delay113/1
  Delay113/1 -> Switch_on68/3, Delay113_enbsw/3
  Delay112_enbsw/1 -> Delay112/1
  Delay112/1 -> Switch_on67/3, Delay112_enbsw/3
  Delay111_enbsw/1 -> Delay111/1
  Delay111/1 -> Switch_on66/3, Delay111_enbsw/3
  Delay110_enbsw/1 -> Delay110/1
  Delay110/1 -> Switch_on65/3, Delay110_enbsw/3
  Delay109_enbsw/1 -> Delay109/1
  Delay109/1 -> Switch_on64/3, Delay109_enbsw/3
  Delay108_enbsw/1 -> Delay108/1
  Delay108/1 -> Switch_on63/3, Delay108_enbsw/3
  Delay107_enbsw/1 -> Delay107/1
  Delay107/1 -> Switch_on62/3, Delay107_enbsw/3
  Delay106_enbsw/1 -> Delay106/1
  Delay106/1 -> Switch_on61/3, Delay106_enbsw/3
  Delay105_enbsw/1 -> Delay105/1
  Delay105/1 -> Switch_on60/3, Delay105_enbsw/3
  Delay104_enbsw/1 -> Delay104/1
  Delay104/1 -> Switch_on59/3, Delay104_enbsw/3
  Delay20/1 -> Switch_on21/3
  Delay19/1 -> Switch_on20/3
  Delay18/1 -> Switch_on19/3
  Delay17/1 -> Switch_on18/3
  Delay16_enbsw/1 -> Delay16/1
  Delay16/1 -> Switch_on17/3, Delay16_enbsw/3
  Delay15_enbsw/1 -> Delay15/1
  Delay15/1 -> Switch_on16/3, Delay15_enbsw/3
  Delay14_enbsw/1 -> Delay14/1
  Delay14/1 -> Switch_on15/3, Delay14_enbsw/3
  Delay13_enbsw/1 -> Delay13/1
  Delay13/1 -> Switch_on13/3, Delay13_enbsw/3
  Delay12/1 -> Switch_on12/3
  Delay11_enbsw/1 -> Delay11/1
  Delay11/1 -> Switch_on11/3, Delay11_enbsw/3
  Delay10/1 -> Switch_on10/3
  Delay9/1 -> Switch_on9/3
  Delay8/1 -> Switch_on8/3

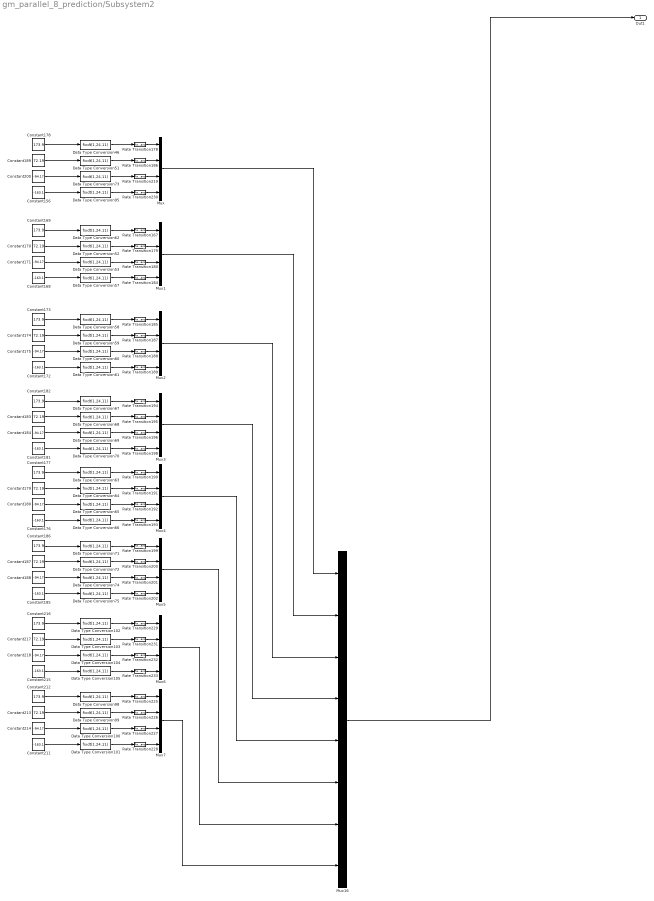
== system gm_parallel_8_prediction/Subsystem2 ==
  Constant{156,168,172,176,181,185,211,215} (8 alike) : Constant  Value=-163.1
  Constant{169,173,177..178,182,186,212,216} (8 alike) : Constant  Value=173.9
  Constant{170,174,179,183,187,189,213,217} (8 alike) : Constant  Value=72.19
  Constant{171,175,180,184,188,200,214,218} (8 alike) : Constant  Value=-94.17
  Data Type Conversion{46,51..53,57..75,95,98..105} (32 alike) : DataTypeConversion  OutDataTypeStr=fixdt(1,24,11)  SaturateOnIntegerOverflow=off  RndMeth=Floor
  Mux{,1..7} (8 alike) : Mux
  Mux16 : Mux  Inputs=8
  Rate Transition{167,178..180,184..196,198..202,219,225..233} (32 alike) : RateTransition  OutPortSampleTime=Rt
  Out1 : Outport
  wires:
  Mux16/1 -> Out1/1
  Data Type Conversion65/1 -> Rate Transition192/1
  Data Type Conversion100/1 -> Rate Transition227/1
  Constant218/1 -> Data Type Conversion104/1
  Constant177/1 -> Data Type Conversion63/1
  Constant183/1 -> Data Type Conversion68/1
  Constant176/1 -> Data Type Conversion66/1
  Data Type Conversion74/1 -> Rate Transition201/1
  Data Type Conversion105/1 -> Rate Transition233/1
  Data Type Conversion104/1 -> Rate Transition232/1
  Constant217/1 -> Data Type Conversion103/1
  Data Type Conversion72/1 -> Rate Transition200/1
  Constant174/1 -> Data Type Conversion59/1
  Rate Transition185/1 -> Mux2/1
  Rate Transition196/1 -> Mux3/3
  Rate Transition230/1 -> Mux/4
  Rate Transition167/1 -> Mux1/1
  Rate Transition219/1 -> Mux/3
  Data Type Conversion102/1 -> Rate Transition229/1
  Constant156/1 -> Data Type Conversion95/1
  Rate Transition198/1 -> Mux3/4
  Rate Transition200/1 -> Mux5/2
  Rate Transition192/1 -> Mux4/3
  Rate Transition190/1 -> Mux4/1
  Constant170/1 -> Data Type Conversion52/1
  Rate Transition195/1 -> Mux3/2
  Data Type Conversion67/1 -> Rate Transition194/1
  Data Type Conversion73/1 -> Rate Transition219/1
  Constant184/1 -> Data Type Conversion69/1
  Rate Transition184/1 -> Mux1/4
  Data Type Conversion70/1 -> Rate Transition198/1
  Constant182/1 -> Data Type Conversion67/1
  Data Type Conversion75/1 -> Rate Transition202/1
  Constant189/1 -> Data Type Conversion51/1
  Data Type Conversion59/1 -> Rate Transition187/1
  Constant172/1 -> Data Type Conversion61/1
  Data Type Conversion57/1 -> Rate Transition184/1
  Data Type Conversion61/1 -> Rate Transition189/1
  Rate Transition231/1 -> Mux6/2
  Constant173/1 -> Data Type Conversion58/1
  Rate Transition189/1 -> Mux2/4
  Rate Transition226/1 -> Mux7/2
  Constant211/1 -> Data Type Conversion101/1
  Constant213/1 -> Data Type Conversion99/1
  Data Type Conversion46/1 -> Rate Transition178/1
  Data Type Conversion63/1 -> Rate Transition190/1
  Constant168/1 -> Data Type Conversion57/1
  Data Type Conversion101/1 -> Rate Transition228/1
  Rate Transition179/1 -> Mux1/2
  Data Type Conversion62/1 -> Rate Transition167/1
  Constant175/1 -> Data Type Conversion60/1
  Rate Transition225/1 -> Mux7/1
  Mux7/1 -> Mux16/8
  Data Type Conversion66/1 -> Rate Transition193/1
  Constant186/1 -> Data Type Conversion71/1
  Data Type Conversion98/1 -> Rate Transition225/1
  Rate Transition178/1 -> Mux/1
  Mux4/1 -> Mux16/5
  Data Type Conversion52/1 -> Rate Transition179/1
  Constant185/1 -> Data Type Conversion75/1
  Constant216/1 -> Data Type Conversion102/1
  Constant214/1 -> Data Type Conversion100/1
  Rate Transition228/1 -> Mux7/4
  Data Type Conversion69/1 -> Rate Transition196/1
  Constant171/1 -> Data Type Conversion53/1
  Rate Transition227/1 -> Mux7/3
  Mux1/1 -> Mux16/2
  Constant215/1 -> Data Type Conversion105/1
  Mux/1 -> Mux16/1
  Data Type Conversion68/1 -> Rate Transition195/1
  Constant178/1 -> Data Type Conversion46/1
  Mux6/1 -> Mux16/7
  Data Type Conversion53/1 -> Rate Transition180/1
  Rate Transition232/1 -> Mux6/3
  Rate Transition186/1 -> Mux/2
  Rate Transition193/1 -> Mux4/4
  Constant212/1 -> Data Type Conversion98/1
  Constant181/1 -> Data Type Conversion70/1
  Rate Transition202/1 -> Mux5/4
  Rate Transition233/1 -> Mux6/4
  Rate Transition188/1 -> Mux2/3
  Constant180/1 -> Data Type Conversion65/1
  Mux5/1 -> Mux16/6
  Rate Transition194/1 -> Mux3/1
  Rate Transition229/1 -> Mux6/1
  Constant188/1 -> Data Type Conversion74/1
  Constant200/1 -> Data Type Conversion73/1
  Constant179/1 -> Data Type Conversion64/1
  Mux2/1 -> Mux16/3
  Rate Transition191/1 -> Mux4/2
  Data Type Conversion99/1 -> Rate Transition226/1
  Constant187/1 -> Data Type Conversion72/1
  Data Type Conversion51/1 -> Rate Transition186/1
  Data Type Conversion71/1 -> Rate Transition199/1
  Rate Transition199/1 -> Mux5/1
  Mux3/1 -> Mux16/4
  Rate Transition180/1 -> Mux1/3
  Data Type Conversion64/1 -> Rate Transition191/1
  Data Type Conversion58/1 -> Rate Transition185/1
  Rate Transition187/1 -> Mux2/2
  Data Type Conversion60/1 -> Rate Transition188/1
  Data Type Conversion103/1 -> Rate Transition231/1
  Rate Transition201/1 -> Mux5/3
  Data Type Conversion95/1 -> Rate Transition230/1
  Constant169/1 -> Data Type Conversion62/1

== system gm_parallel_8_prediction/Prediction_and_cost_function2/Compare To Constant ==
  u : Inport  OutDataTypeStr=fixdt(1,32,0,'DataTypeOverride', 'Off')  SampleTime=1e-08
  Compare : RelationalOperator  Operator=<=  OutDataTypeStr=boolean
  Constant : Constant  DisableCoverage=on  Value=const  OutDataTypeStr=Inherit: Inherit via back propagation  SampleTime=-1
  y : Outport  SampleTime=1e-08
  wires:
  Compare/1 -> y/1
  Constant/1 -> Compare/2
  u/1 -> Compare/1

== system gm_parallel_8_prediction/Prediction_and_cost_function2/Data Type Conversion1 ==
  In1 : Inport
  Data Type Conversion1 : DataTypeConversion  OutDataTypeStr=single  RndMeth=Nearest  SampleTime=1e-08  SaturateOnIntegerOverflow=off
  Data Type Conversion1_pd1 : Delay  DelayLength=6
  Out1 : Outport
  wires:
  In1/1 -> Data Type Conversion1/1
  Data Type Conversion1/1 -> Data Type Conversion1_pd1/1
  Data Type Conversion1_pd1/1 -> Out1/1

== system gm_parallel_8_prediction/Prediction_and_cost_function2/Data Type Conversion10 ==
  In1 : Inport
  Data Type Conversion10 : DataTypeConversion  OutDataTypeStr=single  RndMeth=Nearest  SampleTime=1e-08  SaturateOnIntegerOverflow=off
  Data Type Conversion10_pd1 : Delay  DelayLength=6
  Out1 : Outport
  wires:
  In1/1 -> Data Type Conversion10/1
  Data Type Conversion10/1 -> Data Type Conversion10_pd1/1
  Data Type Conversion10_pd1/1 -> Out1/1

== system gm_parallel_8_prediction/Prediction_and_cost_function2/Data Type Conversion18 ==
  In1 : Inport
  Data Type Conversion18 : DataTypeConversion  OutDataTypeStr=fixdt(1, 18, 11)  RndMeth=Nearest  SampleTime=1e-08  SaturateOnIntegerOverflow=off
  Data Type Conversion18_pd1 : Delay  DelayLength=6
  Out1 : Outport
  wires:
  In1/1 -> Data Type Conversion18/1
  Data Type Conversion18/1 -> Data Type Conversion18_pd1/1
  Data Type Conversion18_pd1/1 -> Out1/1

== system gm_parallel_8_prediction/Prediction_and_cost_function2/Data Type Conversion4 ==
  In1 : Inport
  Data Type Conversion4 : DataTypeConversion  OutDataTypeStr=single  RndMeth=Nearest  SampleTime=1e-08  SaturateOnIntegerOverflow=off
  Data Type Conversion4_pd1 : Delay  DelayLength=6
  Out1 : Outport
  wires:
  In1/1 -> Data Type Conversion4/1
  Data Type Conversion4/1 -> Data Type Conversion4_pd1/1
  Data Type Conversion4_pd1/1 -> Out1/1

== system gm_parallel_8_prediction/Prediction_and_cost_function2/Data Type Conversion7 ==
  In1 : Inport
  Data Type Conversion7 : DataTypeConversion  OutDataTypeStr=single  RndMeth=Nearest  SampleTime=1e-08  SaturateOnIntegerOverflow=off
  Data Type Conversion7_pd1 : Delay  DelayLength=6
  Out1 : Outport
  wires:
  In1/1 -> Data Type Conversion7/1
  Data Type Conversion7/1 -> Data Type Conversion7_pd1/1
  Data Type Conversion7_pd1/1 -> Out1/1

== system gm_parallel_8_prediction/Prediction_and_cost_function2/Data Type Conversion8 ==
  In1 : Inport
  Data Type Conversion8 : DataTypeConversion  OutDataTypeStr=single  RndMeth=Nearest  SampleTime=1e-08  SaturateOnIntegerOverflow=off
  Data Type Conversion8_pd1 : Delay  DelayLength=6
  Out1 : Outport
  wires:
  In1/1 -> Data Type Conversion8/1
  Data Type Conversion8/1 -> Data Type Conversion8_pd1/1
  Data Type Conversion8_pd1/1 -> Out1/1

== system gm_parallel_8_prediction/Prediction_and_cost_function2/Data Type Conversion9 ==
  In1 : Inport
  Data Type Conversion9 : DataTypeConversion  OutDataTypeStr=single  RndMeth=Nearest  SampleTime=1e-08  SaturateOnIntegerOverflow=off
  Data Type Conversion9_pd1 : Delay  DelayLength=6
  Out1 : Outport
  wires:
  In1/1 -> Data Type Conversion9/1
  Data Type Conversion9/1 -> Data Type Conversion9_pd1/1
  Data Type Conversion9_pd1/1 -> Out1/1

== system gm_parallel_8_prediction/Prediction_and_cost_function2/Detect Rise Positive ==
  note: Edge
  note: U(k)
  U : Inport  OutDataTypeStr=boolean  SampleTime=1e-08
  Delay Input1 : UnitDelay  Description=Store in Global RAM  DisableCoverage=on  InitialCondition=vinit  SampleTime=-1  HasFrameUpgradeWarning=on
  FixPt Relational Operator : RelationalOperator  Operator=>  OutDataTypeStr=boolean  ZeroCross=off  InputSameDT=off
  Positive : Subsystem  mask(Compare To Zero){relop=>, OutDataTypeStr=boolean, ZeroCross=off}
      mask prompts: relop "Simulink:masks:Operator_MP"; OutDataTypeStr "Simulink:masks:OutputDataType_MP"; ZeroCross "Simulink:masks:EnableZerocrossingDetection_MP"
      mask help: Simulink:masks:CompareToZero_MD
      mask init:
      | OutDataTypeStr = 'boolean';
      | ZeroCross = 'off';
      | blkName = 'parallel_8_prediction/Prediction_and_cost_function2/Detect Rise\nPositive/Positive';
      | relop = '>';
      | setValue = 'boolean';
      mask TypeOptions relop: == | ~= | < | <= | >= | >
      mask TypeOptions OutDataTypeStr: Simulink:masks:uint8 | Simulink:masks:boolean
      mask Callback ZeroCross: sl('zeroCrossEnable', gcbh);
      mask Display: disp([relop,' 0'])
  Y : Outport  SampleTime=1e-08
  wires:
  Delay Input1/1 -> FixPt Relational Operator/2
  FixPt Relational Operator/1 -> Y/1
  Positive/1(y) -> FixPt Relational Operator/1, Delay Input1/1
  U/1 -> Positive/1(u)

== system gm_parallel_8_prediction/Prediction_and_cost_function2/Detect Rise Positive1 ==
  note: Edge
  note: U(k)
  U : Inport  OutDataTypeStr=boolean  SampleTime=1e-08
  Delay Input1 : UnitDelay  Description=Store in Global RAM  DisableCoverage=on  InitialCondition=vinit  SampleTime=-1  HasFrameUpgradeWarning=on
  FixPt Relational Operator : RelationalOperator  Operator=>  OutDataTypeStr=boolean  ZeroCross=off  InputSameDT=off
  Positive : Subsystem  mask(Compare To Zero){relop=>, OutDataTypeStr=boolean, ZeroCross=off}
      mask prompts: relop "Simulink:masks:Operator_MP"; OutDataTypeStr "Simulink:masks:OutputDataType_MP"; ZeroCross "Simulink:masks:EnableZerocrossingDetection_MP"
      mask help: Simulink:masks:CompareToZero_MD
      mask init:
      | OutDataTypeStr = 'boolean';
      | ZeroCross = 'off';
      | blkName = 'parallel_8_prediction/Prediction_and_cost_function2/Detect Rise\nPositive1/Positive';
      | relop = '>';
      | setValue = 'boolean';
      mask TypeOptions relop: == | ~= | < | <= | >= | >
      mask TypeOptions OutDataTypeStr: Simulink:masks:uint8 | Simulink:masks:boolean
      mask Callback ZeroCross: sl('zeroCrossEnable', gcbh);
      mask Display: disp([relop,' 0'])
  Y : Outport  SampleTime=1e-08
  wires:
  Delay Input1/1 -> FixPt Relational Operator/2
  FixPt Relational Operator/1 -> Y/1
  Positive/1(y) -> FixPt Relational Operator/1, Delay Input1/1
  U/1 -> Positive/1(u)

== system gm_parallel_8_prediction/Prediction_and_cost_function2/Detect Rise Positive2 ==
  note: Edge
  note: U(k)
  U : Inport  OutDataTypeStr=boolean  SampleTime=1e-08
  Delay Input1 : UnitDelay  Description=Store in Global RAM  DisableCoverage=on  InitialCondition=vinit  SampleTime=-1  HasFrameUpgradeWarning=on
  FixPt Relational Operator : RelationalOperator  Operator=>  OutDataTypeStr=boolean  ZeroCross=off  InputSameDT=off
  Positive : Subsystem  mask(Compare To Zero){relop=>, OutDataTypeStr=boolean, ZeroCross=off}
      mask prompts: relop "Simulink:masks:Operator_MP"; OutDataTypeStr "Simulink:masks:OutputDataType_MP"; ZeroCross "Simulink:masks:EnableZerocrossingDetection_MP"
      mask help: Simulink:masks:CompareToZero_MD
      mask init:
      | OutDataTypeStr = 'boolean';
      | ZeroCross = 'off';
      | blkName = 'parallel_8_prediction/Prediction_and_cost_function2/Detect Rise\nPositive2/Positive';
      | relop = '>';
      | setValue = 'boolean';
      mask TypeOptions relop: == | ~= | < | <= | >= | >
      mask TypeOptions OutDataTypeStr: Simulink:masks:uint8 | Simulink:masks:boolean
      mask Callback ZeroCross: sl('zeroCrossEnable', gcbh);
      mask Display: disp([relop,' 0'])
  Y : Outport  SampleTime=1e-08
  wires:
  Delay Input1/1 -> FixPt Relational Operator/2
  FixPt Relational Operator/1 -> Y/1
  Positive/1(y) -> FixPt Relational Operator/1, Delay Input1/1
  U/1 -> Positive/1(u)

== system gm_parallel_8_prediction/Prediction_and_cost_function2/Product ==
  In1 : Inport
  In2 : Inport  Port=2
  Product : Product  Inputs=**  OutDataTypeStr=single  SampleTime=1e-08
  Product_pd1 : Delay  DelayLength=6
  Out1 : Outport
  wires:
  In1/1 -> Product/1
  In2/1 -> Product/2
  Product/1 -> Product_pd1/1
  Product_pd1/1 -> Out1/1
